simulink model "digital8"  (R2024a)
settings: Solver=VariableStepAuto  StartTime=0.0  StopTime=10.0  RelTol=1e-3
settings Model: Creator=tusha  LastModifiedBy=tusha

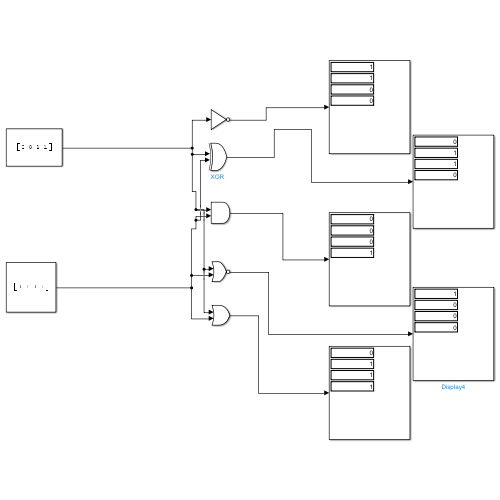
[thumbnail: Simulink's stored preview of the top-level diagram]
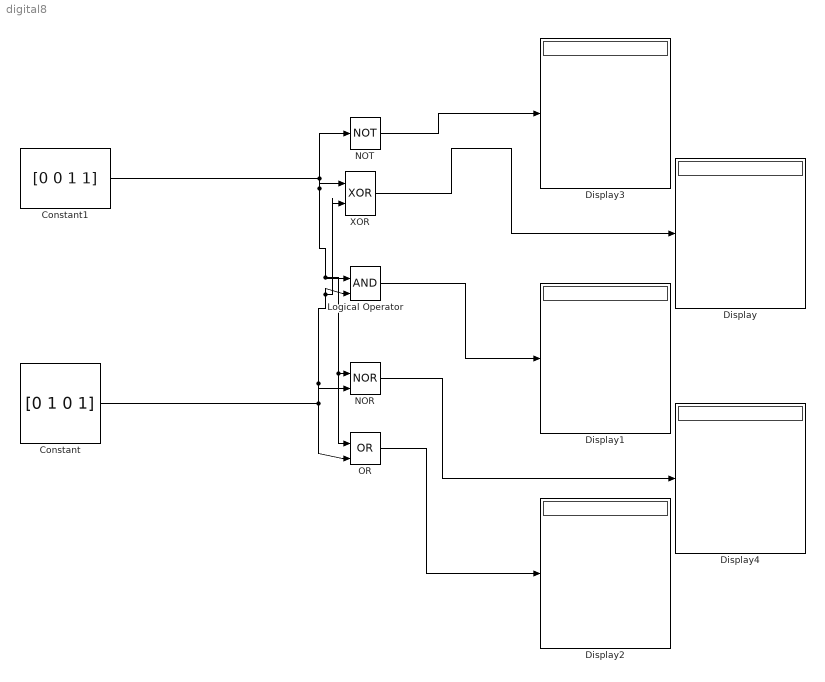
== system digital8 ==
  Constant : Constant  Value=[0 1 0 1]
  Constant1 : Constant  Value=[0 0 1 1]
  Display{,1..4} (5 alike) : Display
  Logical Operator : Logic  IconShape=distinctive  AllPortsSameDT=off  OutDataTypeStr=boolean
  NOR : Logic  Operator=NOR  IconShape=distinctive  AllPortsSameDT=off  OutDataTypeStr=boolean
  NOT : Logic  Operator=NOT  IconShape=distinctive  AllPortsSameDT=off  OutDataTypeStr=boolean
  OR : Logic  Operator=OR  IconShape=distinctive  AllPortsSameDT=off  OutDataTypeStr=boolean
  XOR : Logic  Operator=XOR  IconShape=distinctive  AllPortsSameDT=off  OutDataTypeStr=boolean
  wires:
  Constant/1 -> XOR/2, Logical Operator/2, NOR/2, OR/2
  Constant1/1 -> OR/1, NOR/1, Logical Operator/1, XOR/1, NOT/1
  NOT/1 -> Display3/1
  XOR/1 -> Display/1
  Logical Operator/1 -> Display1/1
  NOR/1 -> Display4/1
  OR/1 -> Display2/1
